simulink model "problem3"  (R2020b)
settings: Solver=VariableStepAuto  StartTime=0.0  StopTime=1  MaxStep=0.0001  RelTol=1e-3
settings Model: Creator=Gopinath Murugan  LastModifiedBy=Gopinath Murugan

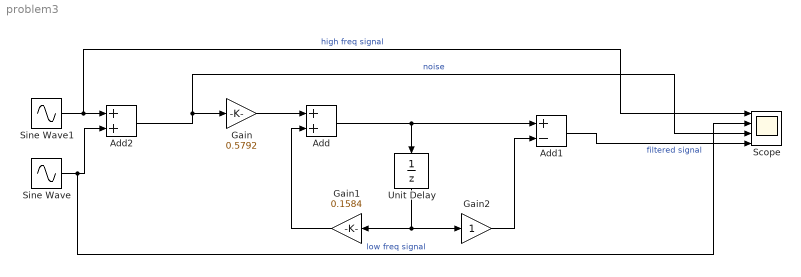
== system problem3 ==
  Add : Sum
  Add1 : Sum  Inputs=+-
  Add2 : Sum
  Gain : Gain  Gain=0.5792
  Gain1 : Gain  Gain=0.1584
  Gain2 : Gain
  Scope : Scope  NumInputPorts=4
  Sine Wave : Sin  Frequency=100  SampleTime=0
  Sine Wave1 : Sin  Frequency=1500  SampleTime=0
  Unit Delay : UnitDelay  SampleTime=-1  HasFrameUpgradeWarning=on
  wires:
  Gain/1 -> Add/1
  Add/1 -> Add1/1, Unit Delay/1
  Unit Delay/1 -> Gain1/1, Gain2/1
  Gain1/1 -> Add/2
  Gain2/1 -> Add1/2
  Add1/1 -> Scope/4  "filtered signal"
  Add2/1 -> Scope/3, Gain/1  "noise"
  Sine Wave1/1 -> Scope/1, Add2/1  "high freq signal"
  Sine Wave/1 -> Scope/2, Add2/2  "low freq signal"
